simulink model "TwoOneThree_allBlock"  (R2022b)
settings: Solver=VariableStepAuto  StartTime=0.0  StopTime=10.0  RelTol=1e-3
settings Model: Creator=yeyi5  LastModifiedBy=yeyi5

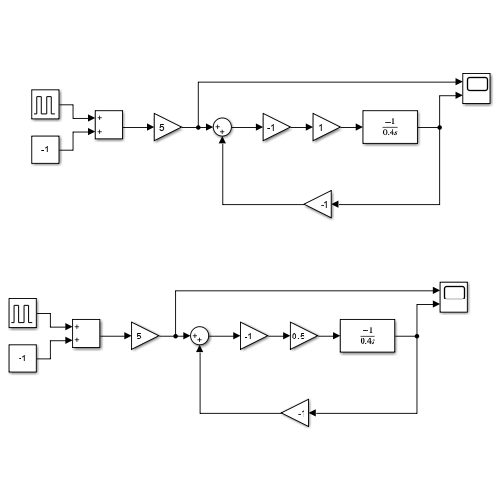
[thumbnail: Simulink's stored preview of the top-level diagram]
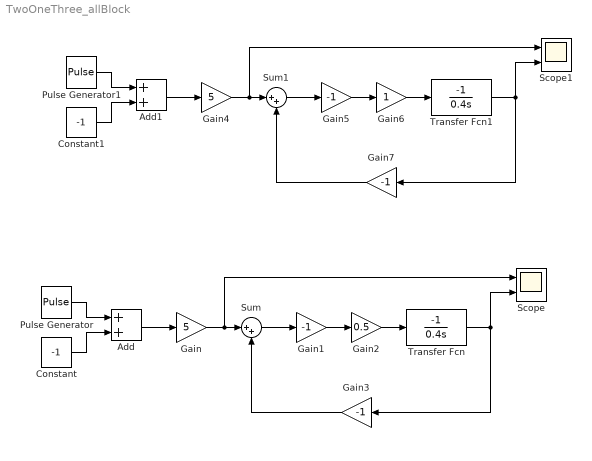
== system TwoOneThree_allBlock ==
  Add : Sum
  Add1 : Sum
  Constant : Constant  Value=-1
  Constant1 : Constant  Value=-1
  Gain : Gain  Gain=5
  Gain{1,3,5,7} (4 alike) : Gain  Gain=-1
  Gain2 : Gain  Gain=0.5
  Gain4 : Gain  Gain=5
  Gain6 : Gain
  Pulse Generator : DiscretePulseGenerator  PulseType=Time based  Amplitude=2  Period=1/0.1  PulseWidth=50
  Pulse Generator1 : DiscretePulseGenerator  PulseType=Time based  Amplitude=2  Period=1/0.1  PulseWidth=50
  Scope : Scope  NumInputPorts=2
  Scope1 : Scope  NumInputPorts=2
  Sum : Sum  Inputs=|++
  Sum1 : Sum  Inputs=|++
  Transfer Fcn : TransferFcn  Numerator=[-1]  Denominator=[0.4 0]
  Transfer Fcn1 : TransferFcn  Numerator=[-1]  Denominator=[0.4 0]
  wires:
  Pulse Generator/1 -> Add/1
  Constant/1 -> Add/2
  Add/1 -> Gain/1
  Gain/1 -> Scope/1, Sum/1
  Sum/1 -> Gain1/1
  Gain1/1 -> Gain2/1
  Gain2/1 -> Transfer Fcn/1
  Gain3/1 -> Sum/2
  Transfer Fcn/1 -> Scope/2, Gain3/1
  Add1/1 -> Gain4/1
  Sum1/1 -> Gain5/1
  Gain6/1 -> Transfer Fcn1/1
  Transfer Fcn1/1 -> Scope1/2, Gain7/1
  Gain5/1 -> Gain6/1
  Gain7/1 -> Sum1/2
  Gain4/1 -> Scope1/1, Sum1/1
  Constant1/1 -> Add1/2
  Pulse Generator1/1 -> Add1/1
